simulink model "Practica1a"  (R2020b)
settings: Solver=VariableStepAuto  StartTime=0.0  StopTime=10.0  RelTol=1e-3
undefined symbols (not defined in the file or in its folder): DiscIntNeverNeededParam, K, R, sigbuilder_block
libraries: simulink x1
settings Model: Creator=Danie  LastModifiedBy=Danie

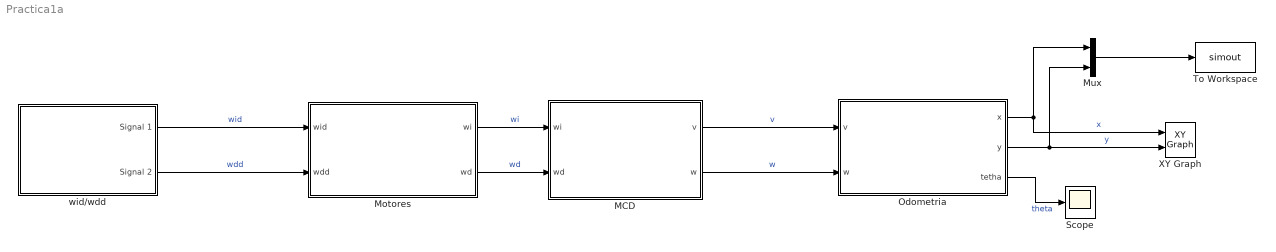
== system Practica1a ==
  MCD : Subsystem
  Motores : Subsystem  mask{kwi=1, kwd=1, twi=0.12, twd=0.12}
  Mux : Mux  Inputs=2
  Odometria : Subsystem
  Scope : Scope
  To Workspace : ToWorkspace  VariableName=simout  SaveFormat=Structure  SampleTime=-1
  XY Graph : simulink/Sinks/XY Graph  xmin=-5  xmax=5  ymin=-5  ymax=5  st=-1
  wid/wdd : Subsystem  Tag=STV Subsys  LoadFcn=sigbuilder_block('load');  StartFcn=sigbuilder_block('start');  StopFcn=sigbuilder_block('stop');  ClipboardFcn=sigbuilder_block('clipboard');  mask(Sigbuilder block){tuvar=[0:10]}
      mask help: Simulink:masks:SigbuilderBlock_MD
      mask init:
      | if ~strcmp(get_param(bdroot(gcbh),'SimulationStatus'),'stopped') tuvar = sigbuilder_block('maskInit'); end
      settings: CopyFcn=sigbuilder_block('copy');  DeleteFcn=sigbuilder_block('delete');  ModelCloseFcn=sigbuilder_block('modelClose');  PreSaveFcn=sigbuilder_block('preSave');  PauseFcn=sigbuilder_block('pause');  ContinueFcn=sigbuilder_block('continue');  NameChangeFcn=sigbuilder_block('namechange');  OpenFcn=sigbuilder_block('open',[422.25 208.5 1152 561.75 ]);  CloseFcn=sigbuilder_block('close');
      mask Display: plot(0, 0, 100, 100,[2, 2, 32, 32, 2], [68, 8, 8, 68, 68],[32, 2], [38, 38], [32, 19, 2],[53, 60, 44], [32, 17, 17, 2],[16, 16, 31, 31]);txt = getActiveGroup(gcbh);text(2, 100, txt,'verticalAlignment', 'top');
  wires:
  Odometria/2(y) -> Mux/2, XY Graph/2  "y"
  Odometria/3(tetha) -> Scope/1  "theta"
  Mux/1 -> To Workspace/1
  MCD/2(w) -> Odometria/2(w)  "w"
  wid/wdd/1(Signal 1) -> Motores/1(wid)  "wid"
  MCD/1(v) -> Odometria/1(v)  "v"
  wid/wdd/2(Signal 2) -> Motores/2(wdd)  "wdd"
  Motores/1(wi) -> MCD/1(wi)  "wi"
  Odometria/1(x) -> XY Graph/1, Mux/1  "x"
  Motores/2(wd) -> MCD/2(wd)  "wd"

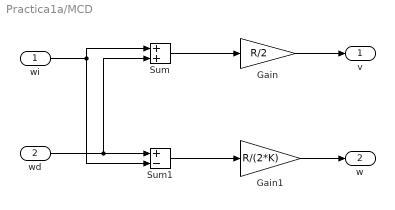
== system Practica1a/MCD ==
  wi : Inport
  wd : Inport  Port=2
  Gain : Gain  Gain=R/2
  Gain1 : Gain  Gain=R/(2*K)
  Sum : Sum
  Sum1 : Sum  Inputs=+-
  v : Outport  VectorParamsAs1DForOutWhenUnconnected=off
  w : Outport  Port=2  VectorParamsAs1DForOutWhenUnconnected=off
  wires:
  Gain/1 -> v/1
  wi/1 -> Sum/1, Sum1/2
  Sum1/1 -> Gain1/1
  wd/1 -> Sum/2, Sum1/1
  Sum/1 -> Gain/1
  Gain1/1 -> w/1

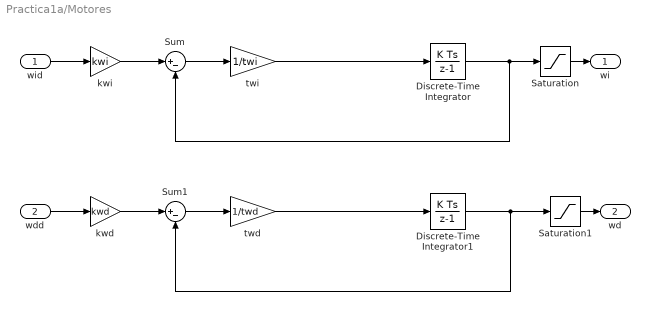
== system Practica1a/Motores ==
  wid : Inport
  wdd : Inport  Port=2
  Discrete-Time Integrator : DiscreteIntegrator  SampleTime=0.025  ICPrevOutput=DiscIntNeverNeededParam  ICPrevScaledInput=DiscIntNeverNeededParam
  Discrete-Time Integrator1 : DiscreteIntegrator  SampleTime=0.025  ICPrevOutput=DiscIntNeverNeededParam  ICPrevScaledInput=DiscIntNeverNeededParam
  Saturation : Saturate  UpperLimit=15  LowerLimit=-15
  Saturation1 : Saturate  UpperLimit=15  LowerLimit=-15
  Sum : Sum  Inputs=|+-
  Sum1 : Sum  Inputs=|+-
  kwd : Gain  Gain=kwd
  kwi : Gain  Gain=kwi
  twd : Gain  Gain=1/twd
  twi : Gain  Gain=1/twi
  wi : Outport  VectorParamsAs1DForOutWhenUnconnected=off
  wd : Outport  Port=2  VectorParamsAs1DForOutWhenUnconnected=off
  wires:
  kwi/1 -> Sum/1
  Discrete-Time Integrator/1 -> Sum/2, Saturation/1
  Sum/1 -> twi/1
  Saturation/1 -> wi/1
  twi/1 -> Discrete-Time Integrator/1
  Discrete-Time Integrator1/1 -> Sum1/2, Saturation1/1
  wid/1 -> kwi/1
  twd/1 -> Discrete-Time Integrator1/1
  kwd/1 -> Sum1/1
  Sum1/1 -> twd/1
  Saturation1/1 -> wd/1
  wdd/1 -> kwd/1

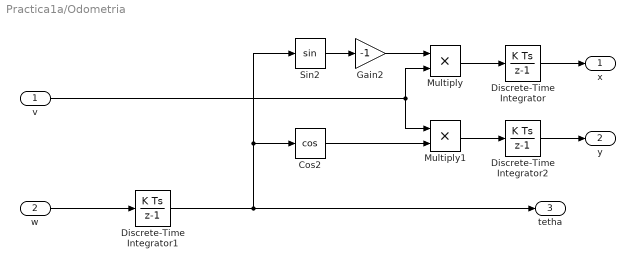
== system Practica1a/Odometria ==
  v : Inport
  w : Inport  Port=2
  Cos2 : Trigonometry  Operator=cos
  Discrete-Time Integrator : DiscreteIntegrator  SampleTime=-1  ICPrevOutput=DiscIntNeverNeededParam  ICPrevScaledInput=DiscIntNeverNeededParam
  Discrete-Time Integrator1 : DiscreteIntegrator  SampleTime=-1  ICPrevOutput=DiscIntNeverNeededParam  ICPrevScaledInput=DiscIntNeverNeededParam
  Discrete-Time Integrator2 : DiscreteIntegrator  SampleTime=-1  ICPrevOutput=DiscIntNeverNeededParam  ICPrevScaledInput=DiscIntNeverNeededParam
  Gain2 : Gain  Gain=-1
  Multiply : Product
  Multiply1 : Product
  Sin2 : Trigonometry
  x : Outport  VectorParamsAs1DForOutWhenUnconnected=off
  y : Outport  Port=2  VectorParamsAs1DForOutWhenUnconnected=off
  tetha : Outport  Port=3  VectorParamsAs1DForOutWhenUnconnected=off
  wires:
  Multiply1/1 -> Discrete-Time Integrator2/1
  Discrete-Time Integrator1/1 -> Cos2/1, Sin2/1, tetha/1
  w/1 -> Discrete-Time Integrator1/1
  v/1 -> Multiply1/1, Multiply/2
  Multiply/1 -> Discrete-Time Integrator/1
  Sin2/1 -> Gain2/1
  Cos2/1 -> Multiply1/2
  Gain2/1 -> Multiply/1
  Discrete-Time Integrator/1 -> x/1
  Discrete-Time Integrator2/1 -> y/1

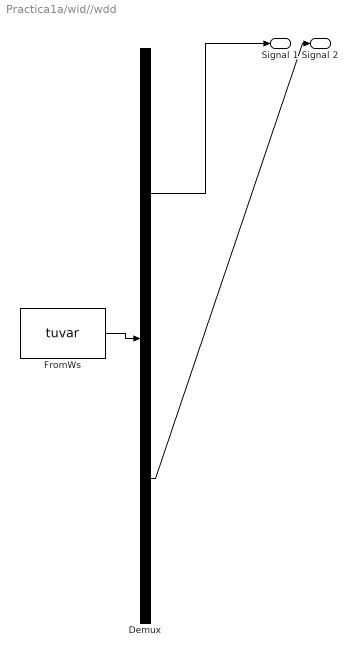
== system Practica1a/wid//wdd ==
  Demux : Demux  Tag=STV Demux  Outputs=2
      settings: DisplayOption=none
  FromWs : FromWorkspace  Tag=STV FromWs  VariableName=tuvar
      SigBuilderData=|
      | common.afterFinalStr = 'Extrapolate'
      | common.sampleTime = 0
      | dataSet.timeRange = [0 30]
      | dataSet.name = 'Group 1'
      | sbobj.Groups.Name = 'Group 1'
      | sbobj.Groups.Signals(1).Name = 'Signal 1'
      | sbobj.Groups.Signals(1).XData = [0 1 1 3.45 3.45 5 5 7 7 13.25 13.25 15 15 25.05 25.05 26.8 26.8 30]
      | sbobj.Groups.Signals(1).YData = [0 0 15 15 0 0 15 15 0 0 -15 -15 0 0 15 15 0 0]
      | sbobj.Groups.Signals(2).Name = 'Signal 2'
      | sbobj.Groups.Signals(2).XData = [0 1 1 3.3 3.3 13.2 13.2 15 15 18.2 18.2 20 20 25.05 25.05 26.9 26.9 30]
      | sbobj.Groups.Signals(2).YData = [0 0 15 15 0 0 15 15 0 0 15 15 0 0 15 15 0 0]
      | sbobj.Groups.TimeRange = [0 30]
  Signal 1 : Outport  Tag=STV Outport  VectorParamsAs1DForOutWhenUnconnected=off
  Signal 2 : Outport  Tag=STV Outport  Port=2  VectorParamsAs1DForOutWhenUnconnected=off
  wires:
  Demux/2 -> Signal 2/1
  FromWs/1 -> Demux/1
  Demux/1 -> Signal 1/1
